simulink model "ATTN"  (R2023a)
settings: Solver=FixedStepAuto  StartTime=0.0  StopTime=40000  RelTol=1e-3
model workspace (MAT data in the model file):
  SampleTime = 0.001
  T_npxls = 4
  T_pupil = 100
  T_whisk = 20
  maxFrame = 3600000
  rewardDuration = 0.05
  targetSide = 1
  toneDuration = 1.5
  trainingStage = 3
  triangleAmplitude = 10
  triangleDuration = 0.1
undefined symbols (not defined in the file or in its folder): Ended, fdesignblkfcn, gcbh, Single
libraries: speedgoatlib_IO191 x5
(part 3 of 3)

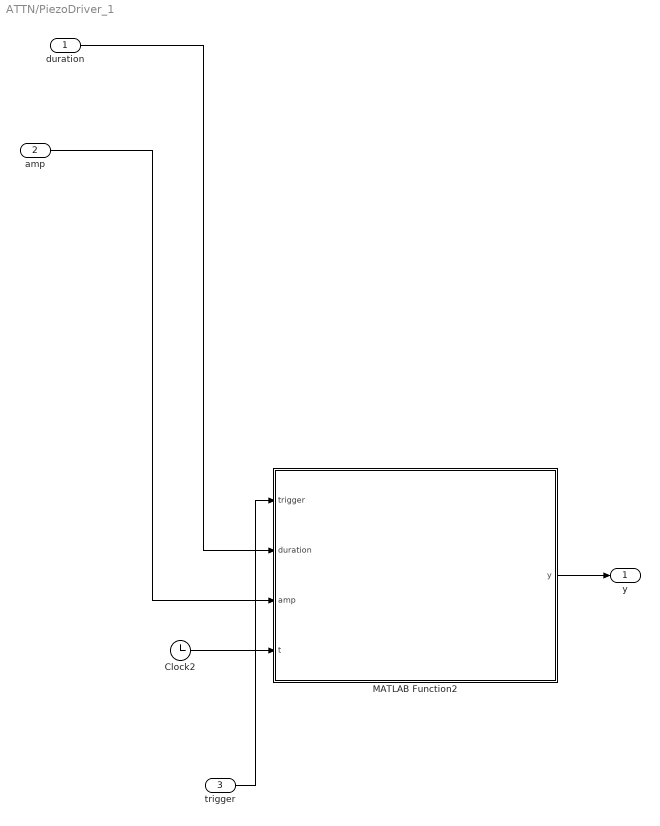
== system ATTN/PiezoDriver_1 ==
  duration : Inport
  amp : Inport  Port=2
  trigger : Inport  Port=3
  Clock2 : Clock
  MATLAB Function2 : MATLAB Function  TreatAsAtomicUnit=on
  y : Outport
  wires:
  Clock2/1 -> MATLAB Function2/4(t)
  MATLAB Function2/1(y) -> y/1
  amp/1 -> MATLAB Function2/3(amp)
  trigger/1 -> MATLAB Function2/1(trigger)
  duration/1 -> MATLAB Function2/2(duration)

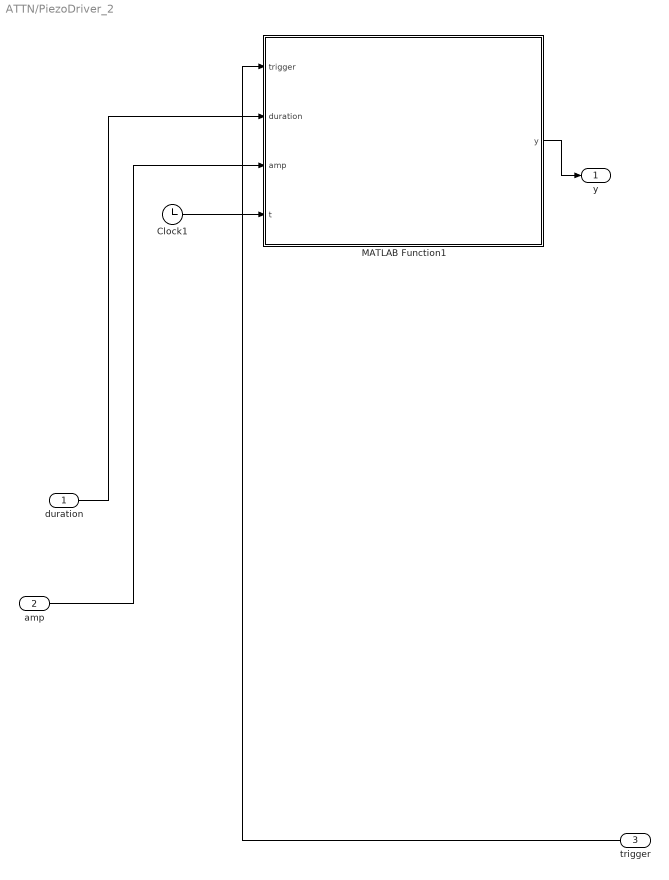
== system ATTN/PiezoDriver_2 ==
  duration : Inport
  amp : Inport  Port=2
  trigger : Inport  Port=3
  Clock1 : Clock
  MATLAB Function1 : MATLAB Function  TreatAsAtomicUnit=on
  y : Outport
  wires:
  Clock1/1 -> MATLAB Function1/4(t)
  trigger/1 -> MATLAB Function1/1(trigger)
  amp/1 -> MATLAB Function1/3(amp)
  duration/1 -> MATLAB Function1/2(duration)
  MATLAB Function1/1(y) -> y/1

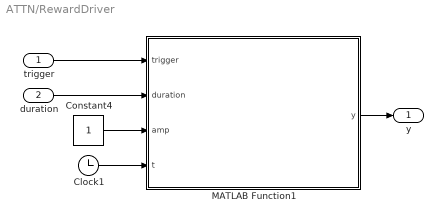
== system ATTN/RewardDriver ==
  trigger : Inport
  duration : Inport  Port=2
  Clock1 : Clock
  Constant4 : Constant  SampleTime=SampleTime
  MATLAB Function1 : MATLAB Function  TreatAsAtomicUnit=on
  y : Outport
  wires:
  Clock1/1 -> MATLAB Function1/4(t)
  Constant4/1 -> MATLAB Function1/3(amp)
  duration/1 -> MATLAB Function1/2(duration)
  trigger/1 -> MATLAB Function1/1(trigger)
  MATLAB Function1/1(y) -> y/1

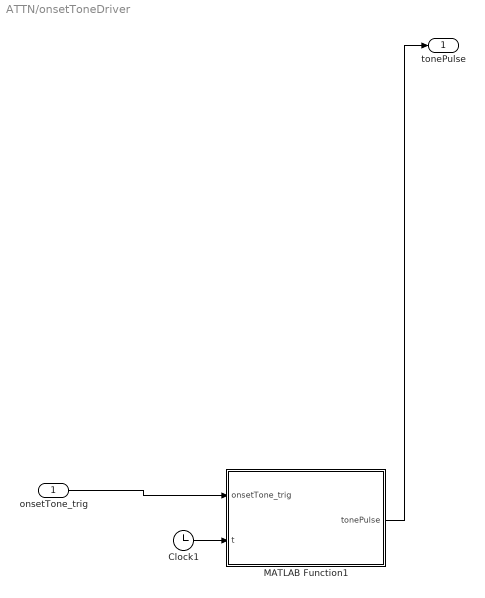
== system ATTN/onsetToneDriver ==
  onsetTone_trig : Inport
  Clock1 : Clock
  MATLAB Function1 : MATLAB Function  TreatAsAtomicUnit=on
  tonePulse : Outport
  wires:
  Clock1/1 -> MATLAB Function1/2(t)
  MATLAB Function1/1(tonePulse) -> tonePulse/1
  onsetTone_trig/1 -> MATLAB Function1/1(onsetTone_trig)

== matlab function ATTN/PiezoDriver_2/MATLAB Function1 ==
  data: trigger input; duration input; amp input; y output; t input
function y = drivePiezo(trigger, duration, amp, t) 
    % When the trigger is received, drivePiezo starts to output a triangle 
    % wave defined by duration and amplitude
    
    % If the trigger is not received, it checks whether t0 is not 
    % empty (indicating that a trigger has been received previously). 
    % If t0 is not empty, it checks if (t - t0) is less than 1.5 seconds. 
    % If so, it keeps tonePulse set to 1, maintaining the tone pulse for 
    % 1.5 seconds after the trigger. 
      
    
    persistent t0;
    persistent y0;
    increment = amp / (duration*1000/2);

    if trigger                
        t0 = t; % store current time 
        y = 0;
        y0 = y;
    elseif ~isempty(t0) 
        if (t - t0) <= duration/2
            y = y0 + increment;
            y0 = y;
        elseif (t - t0) <= duration
            y = y0 - increment;
            y = max([0,y]);
            y0 = y;
        else
            y = 0;
            clear t0 y0 % reset t0 to initial condition
        end        
    else % reset to 0 if no more trigger activity
        y = 0;        
    end

== matlab function ATTN/RewardDriver/MATLAB Function1 ==
  data: trigger input; y output; duration input; amp input; t input
function y = driveSpout(trigger, duration, amp, t) 
    % When the trigger is received, driveSpout starts to output a square
    % pulse defined by duration and amplitude
    
    % If the trigger is not received, it checks whether t0 is not 
    % empty (indicating that a trigger has been received previously). 
    % If t0 is not empty, it checks if (t - t0) is less than 1.5 seconds. 
    % If so, it keeps tonePulse set to 1, maintaining the tone pulse for 
    % 1.5 seconds after the trigger. 
      
    
    persistent t0;

    if trigger                     
        t0 = t; % store current time 
        y = amp;
    elseif ~isempty(t0) 
        if (t - t0) <= duration
            y = amp;
        else
            y = 0;
            clear t0 % reset t0 to initial condition
        end        
    else % reset to 0 if no more trigger activity
        y = 0;        
    end
end

== matlab function ATTN/MATLAB Function1 ==
  data: ADIn input; Lick output; y1 output; Thrd input; x1 input; x2 input; y2 output
function [Lick, y1, y2] = LickDetector(ADIn, Thrd, x1, x2)
%#codegen

ADIn = abs(ADIn);
if x1 == 0
    y1 = 0;
end


if ADIn > Thrd
    y1 = x1+1;
    y2 = x2;
else
    y1 = 0;
    y2 = 0;
end

if (y1 >20) && (x2 == 0)
    Lick =1;
    y2 = 1;
else
    Lick = 0;
%    y2 = x2;
end

== matlab function ATTN/MATLAB Function ==
  data: state_in input; localTime_in input; trialNum_in input; lick input; sessionTime input; npxlsAcq_in input; state_out output; localTime_out output; trialNum_out output; npxlsAcq_out output; counter_in input; numLicks_in input; delay_in input; right_trigger_in input; left_trigger_in input; sampleTime input; counter_out output; numLicks_out output; reward_trigger_out output; right_trigger_out output; left_trigger_out output; delay_out output; was_target_in input; was_target_out output; target_side input; reward_duration_in input; stim_duration_in input; stage input; reward_duration_out output; stim_duration_out output; onsetTone_trig output
function [state_out, localTime_out, trialNum_out, ...
    npxlsAcq_out, counter_out, numLicks_out, reward_trigger_out, ...
    right_trigger_out, left_trigger_out, delay_out, was_target_out, ... 
    reward_duration_out, stim_duration_out, onsetTone_trig] ...
    = nCORTEx(state_in, localTime_in, trialNum_in, lick, ...
    sessionTime, npxlsAcq_in, counter_in, numLicks_in, delay_in, ... 
    right_trigger_in, left_trigger_in, sampleTime, was_target_in, ...
    target_side, reward_duration_in, stim_duration_in, stage)
% stages: 1 - classical conditioning, 2 - opreant conditioning, 3 - impulse
% control, 111 - calibrate reward delivery; 222 - position piezo; 333 -
% calibrate piezo driver triangle duration 
    
    counter_out=counter_in+1;

    switch (stage)
        case {1} %% classical conditioning 
            switch (state_in)         
                % case {0} % LOAD SESSION PARAMS
                    % params = loadSlParams;
                    % state_out = 1;
                case {1} %% TRIAL START
                    npxlsAcq_out=1;
                    state_out = 2; % go to ITI
                    localTime_out = 1;
                    trialNum_out = 1;
                    % reset piezo triggers and lick counter
                    right_trigger_out = 0; % reset piezo triggers 
                    left_trigger_out = 0;
                    numLicks_out = 0;
                    delay_out = sessionTime + negative_exp_rand(5,9);
                    disp('End of ITI')
                    disp(delay_out)
                    reward_trigger_out = 0;
                    was_target_out = 0;
                    reward_duration_out = reward_duration_in;
                    stim_duration_out = stim_duration_in;
                    onsetTone_trig = 0;
        
                case {2} %% inter-trial interval  
                    if sessionTime < delay_in
                        state_out = state_in; % continue with ITI 
                    else
                        state_out = 3; % go to stimulus 
                    end
                    localTime_out = localTime_in + 1;
                    trialNum_out = trialNum_in + 1;
                    npxlsAcq_out=npxlsAcq_in;
                    right_trigger_out = right_trigger_in; % keep piezo triggers 
                    left_trigger_out = left_trigger_in;
                    numLicks_out = numLicks_in;
                    delay_out = delay_in;
                    reward_trigger_out = 0;
                    was_target_out = was_target_in;
                    reward_duration_out = reward_duration_in;
                    stim_duration_out = stim_duration_in;
                    onsetTone_trig = 0;
        
                case {3} %% stimulus onset 
                    if rand() <= 0.8 % 80% distractor stims 
                        if target_side % 1: left target
                            right_trigger_out = 1;
                            left_trigger_out = 0;
                        else % 0: right target
                            left_trigger_out = 1;
                            right_trigger_out = 0;
                        end
                        disp('Distractor')
                        disp(sessionTime)
                        was_target_out = 0;
                    else % 20% target stims 
                        if target_side % 1: left target
                            left_trigger_out = 1;
                            right_trigger_out = 0;
                        else
                            right_trigger_out = 1;
                            left_trigger_out = 0;
                        end
                        disp('Target')
                        disp(sessionTime)
                        was_target_out = 1;
                    end
                    % trigger a piezo  
                    state_out = 4; % go to lockout window
                    delay_out = sessionTime + 0.2;
                    disp('End of lockout')
                    disp(delay_out)
                    localTime_out = localTime_in + 1;
                    trialNum_out = trialNum_in + 1;
                    npxlsAcq_out=npxlsAcq_in;
                    numLicks_out = numLicks_in;
                    reward_trigger_out = 0;
                    reward_duration_out = reward_duration_in;
                    stim_duration_out = stim_duration_in;
                    onsetTone_trig = 0;
        
                case {4} %% lockout window 
                    if sessionTime < delay_in 
                        state_out = state_in;
                        delay_out = delay_in;
                    elseif was_target_in
                        state_out = 5; % deliver reward 
                        delay_out = sessionTime + 1.0;
                    else
                        state_out = 6; % jump to response window (unrewarded)
                        delay_out = sessionTime + 1.0;
                    end
                    localTime_out = localTime_in + 1;
                    trialNum_out = trialNum_in + 1;
                    npxlsAcq_out=npxlsAcq_in;
                    left_trigger_out = 0; % reset piezo triggers
                    right_trigger_out = 0;
                    numLicks_out = numLicks_in;
                    reward_trigger_out = 0;
                    was_target_out = was_target_in;
                    reward_duration_out = reward_duration_in;
                    stim_duration_out = stim_duration_in;
                    onsetTone_trig = 0;
             
                case {5} %% reward delivery `
                    % trigger reward 
                    reward_trigger_out = 1;
                    disp('Deliver Reward')
                    disp(sessionTime)
                    state_out = 6; % go to response window
                    delay_out = delay_in;
                    localTime_out = localTime_in + 1;
                    trialNum_out = trialNum_in + 1;
                    npxlsAcq_out=npxlsAcq_in;
                    numLicks_out = numLicks_in;
                    right_trigger_out = right_trigger_in;
                    left_trigger_out = left_trigger_in;
                    was_target_out = was_target_in;
                    reward_duration_out = reward_duration_in;
                    stim_duration_out = stim_duration_in;
                    onsetTone_trig = 0;

                case {6} %% response window 
                    if sessionTime < delay_in
                        state_out = state_in;
                    else
                        state_out = 1; % start new trial
                        disp('Start new trial')
                        disp(sessionTime)
                    end
                    localTime_out = localTime_in + 1;
                    trialNum_out = trialNum_in + 1;
                    npxlsAcq_out=npxlsAcq_in;
                    numLicks_out = numLicks_in;
                    right_trigger_out = right_trigger_in;
                    left_trigger_out = left_trigger_in;
                    delay_out = delay_in;
                    reward_trigger_out = 0;
                    was_target_out = was_target_in;
                    reward_duration_out = reward_duration_in;
                    stim_duration_out = stim_duration_in;
                    onsetTone_trig = 0;

                otherwise
                    state_out = state_in;
                    localTime_out = localTime_in;
                    trialNum_out = trialNum_in;
                    npxlsAcq_out=npxlsAcq_in;
                    right_trigger_out = right_trigger_in; % reset piezo triggers 
                    left_trigger_out = left_trigger_in;
                    numLicks_out = numLicks_in;
                    delay_out = delay_in;
                    reward_trigger_out = 0;
                    was_target_out = was_target_in;
                    reward_duration_out = reward_duration_in;
                    stim_duration_out = stim_duration_in;
                    onsetTone_trig = 0;
            end
        case {2} %% operant conditioning 
            switch (state_in)         
                % case {0} % LOAD SESSION PARAMS
                    % params = loadSlParams;
                    % state_out = 1;
                
                case {1} %% TRIAL START
                    npxlsAcq_out=1;
                    state_out = 2; % go to ITI
                    localTime_out = 1;
                    trialNum_out = 1;
                    % reset piezo triggers and lick counter
                    right_trigger_out = 0; % reset piezo triggers 
                    left_trigger_out = 0;
                    numLicks_out = 0;
                    delay_out = sessionTime + negative_exp_rand(5,9);
                    disp('End of ITI')
                    disp(delay_out)
                    reward_trigger_out = 0;
                    was_target_out = was_target_in;
                    reward_duration_out = reward_duration_in;
                    stim_duration_out = stim_duration_in;
                    onsetTone_trig = 0;

                case {2} %% inter-trial interval  
                    if sessionTime < delay_in
                        state_out = state_in; % continue with ITI 
                    else
                        state_out = 3; % go to stimulus 
                    end
                    localTime_out = localTime_in + 1;
                    trialNum_out = trialNum_in + 1;
                    npxlsAcq_out=npxlsAcq_in;
                    right_trigger_out = right_trigger_in; % keep piezo triggers 
                    left_trigger_out = left_trigger_in;
                    numLicks_out = numLicks_in;
                    delay_out = delay_in;
                    reward_trigger_out = 0;
                    was_target_out = was_target_in;
                    reward_duration_out = reward_duration_in;
                    stim_duration_out = stim_duration_in;
                    onsetTone_trig = 0;

                case {3} %% stimulus onset 
                    if rand() <= 0.8% distractor stims 
                        if target_side % 1: left target 
                            right_trigger_out = 1;
                            left_trigger_out = 0;
                        else % 0: right target 
                            left_trigger_out = 1;
                            right_trigger_out = 0;
                        end
                        disp('Distractor')
                        disp(sessionTime)
                        was_target_out = 0;
                    else % 20% target stims 
                        if target_side % 1: left target 
                            left_trigger_out = 1;
                            right_trigger_out = 0;
                        else % 0: right target 
                            right_trigger_out = 1;
                            left_trigger_out = 0;
                        end
                        disp('Target')
                        disp(sessionTime)
                        was_target_out = 1;
                    end
                    % trigger a piezo  
                    state_out = 4; % go to lockout window
                    delay_out = sessionTime + 0.2;
                    disp('End of lockout')
                    disp(delay_out)
                    localTime_out = localTime_in + 1;
                    trialNum_out = trialNum_in + 1;
                    npxlsAcq_out=npxlsAcq_in;
                    numLicks_out = numLicks_in;
                    reward_trigger_out = 0;
                    reward_duration_out = reward_duration_in;
                    stim_duration_out = stim_duration_in;
                    onsetTone_trig = 0;

                case {4} %% lockout window 
                    if sessionTime < delay_in 
                        state_out = state_in;
                        delay_out = delay_in;
                    else %if was_target_in
                        state_out = 5; % response window
                        delay_out = sessionTime + 1.5;
                    % else
                    %     state_out = 7; % jump to response window (unrewarded)
                    %     delay_out = sessionTime + 1.0;                   
                    end
                    localTime_out = localTime_in + 1;
                    trialNum_out = trialNum_in + 1;
                    npxlsAcq_out=npxlsAcq_in;
                    numLicks_out = numLicks_in;
                    reward_trigger_out = 0;
                    left_trigger_out = 0; % reset piezo targets 
                    right_trigger_out = 0;
                    was_target_out = was_target_in;
                    reward_duration_out = reward_duration_in;
                    stim_duration_out = stim_duration_in;
                    onsetTone_trig = 0;

                case {5} %% response window 
                    % increment numLicks based on lickometer input 
                    if lick
                        numLicks_out = numLicks_in + 1;
                    else
                        numLicks_out = numLicks_in;
                    end

                    if sessionTime < delay_in
                        state_out = state_in;
                    elseif numLicks_in && was_target_in
                        state_out = 6; % deliver reward
                    else
                        state_out = 1; % start new trial
                        disp('No response')
                        disp(left_trigger_in)
                    end
                    localTime_out = localTime_in + 1;
                    trialNum_out = trialNum_in + 1;
                    npxlsAcq_out=npxlsAcq_in;
                    right_trigger_out = right_trigger_in;
                    delay_out = delay_in;
                    reward_trigger_out = 0;
                    left_trigger_out = left_trigger_in;
                    was_target_out = was_target_in;
                    reward_duration_out = reward_duration_in;
                    stim_duration_out = stim_duration_in;
                    onsetTone_trig = 0;

                case {6} %% reward delivery 
                    % trigger reward 
                    reward_trigger_out = 1;
                    disp('Deliver Reward')
                    disp(sessionTime)
                    state_out = 7; % go to response window
                    delay_out = sessionTime + 0.5;
                    disp('Reward collection')
                    disp(delay_out)
                    localTime_out = localTime_in + 1;
                    trialNum_out = trialNum_in + 1;
                    npxlsAcq_out=npxlsAcq_in;
                    numLicks_out = numLicks_in;
                    right_trigger_out = right_trigger_in;
                    left_trigger_out = left_trigger_in;
                    was_target_out = was_target_in;
                    reward_duration_out = reward_duration_in;
                    stim_duration_out = stim_duration_in;
                    onsetTone_trig = 0;

                case {7} %% reward collection
                    if sessionTime < delay_in
                        state_out = state_in;
                    else
                        state_out = 1; %start new trial
                    end
                    localTime_out = localTime_in + 1;
                    trialNum_out = trialNum_in + 1;
                    npxlsAcq_out=npxlsAcq_in;
                    left_trigger_out = left_trigger_in;
                    right_trigger_out = right_trigger_in;
                    numLicks_out = numLicks_in;
                    delay_out = delay_in;
                    reward_trigger_out = 0;
                    was_target_out = was_target_in;
                    reward_duration_out = reward_duration_in;
                    stim_duration_out = stim_duration_in;
                    onsetTone_trig = 0;

                otherwise
                    state_out = state_in;
                    localTime_out = localTime_in;
                    trialNum_out = trialNum_in;
                    npxlsAcq_out=npxlsAcq_in;
                    left_trigger_out = left_trigger_in;
                    right_trigger_out = right_trigger_in;
                    numLicks_out = numLicks_in;
                    delay_out = delay_in;
                    reward_trigger_out = 0;
                    was_target_out = was_target_in;
                    reward_duration_out = reward_duration_in;
                    stim_duration_out = stim_duration_in;
                    onsetTone_trig = 0;
            end
        case {3} %% impulse control
            switch (state_in)         
                % case {0} % LOAD SESSION PARAMS
                    % params = loadSlParams;
                    % state_out = 1;
                case {1} %% TRIAL START
                    npxlsAcq_out=1;
                    state_out = 2; % go to ITI
                    localTime_out = 1;
                    trialNum_out = 1;
                    % reset piezo triggers and lick counter
                    right_trigger_out = 0; % reset piezo triggers 
                    left_trigger_out = 0;
                    if ~was_target_in && ~numLicks_in 
                        disp('CR')
                        delay_out = sessionTime + negative_exp_rand(2,4);
                    else
                        delay_out = sessionTime + negative_exp_rand(5,9);
                    end
                    numLicks_out = 0;
                    disp('End of ITI')
                    disp(delay_out)
                    reward_trigger_out = 0;
                    was_target_out = 0;
                    reward_duration_out = reward_duration_in;
                    stim_duration_out = stim_duration_in;
                    onsetTone_trig = 0;

                case {2} %% inter-trial interval  
                    if sessionTime < delay_in
                        state_out = state_in; % continue with ITI 
                    else
                        state_out = 3; % go to stimulus 
                    end
                    localTime_out = localTime_in + 1;
                    trialNum_out = trialNum_in + 1;
                    npxlsAcq_out=npxlsAcq_in;
                    right_trigger_out = right_trigger_in; % keep piezo triggers 
                    left_trigger_out = left_trigger_in;
                    numLicks_out = numLicks_in;
                    delay_out = delay_in;
                    reward_trigger_out = 0;
                    was_target_out = was_target_in;
                    reward_duration_out = reward_duration_in;
                    stim_duration_out = stim_duration_in;
                    onsetTone_trig = 0;

                case {3} %% stimulus onset 
                    if rand() <= 0.8 % 80% distractor stims 
                        if target_side % 1: target left
                            right_trigger_out = 1;
                            left_trigger_out = 0;
                        else % 0: target right
                            left_trigger_out = 1;
                            right_trigger_out = 0;
                        end
                        disp('Distractor')
                        disp(sessionTime)
                        was_target_out = 0;
                    else % 20% target stims 
                        if target_side % 1: target left
                            left_trigger_out = 1;
                            right_trigger_out = 0;
                        else % 0: target right
                            right_trigger_out = 1;
                            left_trigger_out = 0;
                        end
                        disp('Target')
                        disp(sessionTime)
                        was_target_out = 1;
                    end
                    % trigger a piezo  
                    state_out = 4; % go to lockout window
                    delay_out = sessionTime + 0.2;
                    disp('End of lockout')
                    disp(delay_out)
                    localTime_out = localTime_in + 1;
                    trialNum_out = trialNum_in + 1;
                    npxlsAcq_out=npxlsAcq_in;
                    numLicks_out = numLicks_in;
                    reward_trigger_out = 0;
                    reward_duration_out = reward_duration_in;
                    stim_duration_out = stim_duration_in;
                    onsetTone_trig = 0;

                case {4} %% lockout window 
                    if sessionTime < delay_in 
                        state_out = state_in;
                        delay_out = delay_in;
                    else %if was_target_in
                        state_out = 5; % response window
                        delay_out = sessionTime + 1.0;
                    % else
                    %     state_out = 7; % jump to response window (unrewarded)
                    %     delay_out = sessionTime + 1.0;                   
                    end
                    localTime_out = localTime_in + 1;
                    trialNum_out = trialNum_in + 1;
                    npxlsAcq_out=npxlsAcq_in;
                    numLicks_out = numLicks_in;
                    reward_trigger_out = 0;
                    left_trigger_out = 0;
                    right_trigger_out = 0;
                    was_target_out = was_target_in;
                    reward_duration_out = reward_duration_in;
                    stim_duration_out = stim_duration_in;
                    onsetTone_trig = 0;

                case {5} %% response window 
                    % increment numLicks based on lickometer input 
                    if was_target_in && rand() < 0.2
                        numLicks_out = numLicks_in + 1;
                    elseif ~was_target_in  && rand() < 0.001
                        numLicks_out = numLicks_in + 1;
                        disp('Licked for distractor')
                    else
                        numLicks_out = numLicks_in;
                    end

                    if sessionTime < delay_in
                        state_out = state_in;
                    elseif numLicks_in && was_target_in
                        state_out = 6; % deliver reward
                    else
                        state_out = 1; % start new trial
                        disp('No response')
                        disp(left_trigger_in)
                    end
                    localTime_out = localTime_in + 1;
                    trialNum_out = trialNum_in + 1;
                    npxlsAcq_out=npxlsAcq_in;
                    right_trigger_out = right_trigger_in;
                    delay_out = delay_in;
                    reward_trigger_out = 0;
                    left_trigger_out = left_trigger_in;
                    was_target_out = was_target_in;
                    reward_duration_out = reward_duration_in;
                    stim_duration_out = stim_duration_in;
                    onsetTone_trig = 0;

                case {6} %% reward delivery 
                    % trigger reward 
                    reward_trigger_out = 1;
                    disp('Deliver Reward')
                    disp(sessionTime)
                    state_out = 7; % go to response window
                    delay_out = sessionTime + 0.5;
                    disp('Reward collection')
                    disp(delay_out)
                    localTime_out = localTime_in + 1;
                    trialNum_out = trialNum_in + 1;
                    npxlsAcq_out=npxlsAcq_in;
                    numLicks_out = numLicks_in;
                    right_trigger_out = right_trigger_in;
                    left_trigger_out = left_trigger_in;
                    was_target_out = was_target_in;
                    reward_duration_out = reward_duration_in;
                    stim_duration_out = stim_duration_in;
                    onsetTone_trig = 0;

                case {7} %% reward collection
                    if sessionTime < delay_in
                        state_out = state_in;
                    else
                        state_out = 1; %start new trial
                    end
                    localTime_out = localTime_in + 1;
                    trialNum_out = trialNum_in + 1;
                    npxlsAcq_out=npxlsAcq_in;
                    left_trigger_out = left_trigger_in;
                    right_trigger_out = right_trigger_in;
                    numLicks_out = numLicks_in;
                    delay_out = delay_in;
                    reward_trigger_out = 0;
                    was_target_out = was_target_in;
                    reward_duration_out = reward_duration_in;
                    stim_duration_out = stim_duration_in;
                    onsetTone_trig = 0;

                otherwise
                    state_out = state_in;
                    localTime_out = localTime_in;
                    trialNum_out = trialNum_in;
                    npxlsAcq_out=npxlsAcq_in;
                    left_trigger_out = left_trigger_in;
                    right_trigger_out = right_trigger_in;
                    numLicks_out = numLicks_in;
                    delay_out = delay_in;
                    reward_trigger_out = 0;
                    was_target_out = was_target_in;
                    reward_duration_out = reward_duration_in;
                    stim_duration_out = stim_duration_in;
                    onsetTone_trig = 0;
            end
        case {111} % calibrate reward delivery 
            switch (state_in)         
                % case {0} % LOAD SESSION PARAMS
                    % params = loadSlParams;
                    % state_out = 1;
                case {1} %% TRIAL START
                    npxlsAcq_out=0;
                    localTime_out = 1;
                    trialNum_out = 1;
                    right_trigger_out = 0; % reset piezo triggers 
                    left_trigger_out = 0;
                    delay_out = sessionTime + 10;
                    numLicks_out = 0;
                    disp(sessionTime)
                    reward_trigger_out = 1;
                    was_target_out = 0;
                    reward_duration_out = 0.02;
                    disp(reward_duration_out)
                    state_out = 2; % go to ITI
                    stim_duration_out = stim_duration_in;
                    onsetTone_trig = 0;

                otherwise
                    if sessionTime < delay_in
                        state_out = state_in;
                        reward_trigger_out = 0;
                        delay_out = delay_in;
                        % reward_duration_out = (state_out-1) * 0.05;
                        reward_duration_out = 0.02;
                    else
                        state_out = state_in + 1; %start new trial
                        reward_trigger_out = 1;
                        delay_out = sessionTime + 10;
                        disp(sessionTime)
                        % reward_duration_out = state_out * 0.01;
                        reward_duration_out = 0.02;
                        disp(reward_duration_out)
                    end
                    localTime_out = localTime_in + 1;
                    trialNum_out = trialNum_in + 1;
                    npxlsAcq_out=npxlsAcq_in;
                    left_trigger_out = left_trigger_in;
                    right_trigger_out = right_trigger_in;
                    numLicks_out = numLicks_in;
                    was_target_out = was_target_in;
                    stim_duration_out = stim_duration_in;
                    onsetTone_trig = 0;
            end

        case {222} % piezo positioning, 1 target stim every 10 s
            switch (state_in)         
                % case {0} % LOAD SESSION PARAMS
                    % params = loadSlParams;
                    % state_out = 1;
                case {1} %% TRIAL START
                    npxlsAcq_out=0;
                    localTime_out = 1;
                    trialNum_out = 1;
                    if target_side % 1: target left
                        right_trigger_out = 1;
                        left_trigger_out = 0;
                    else % 0: target right
                        left_trigger_out = 1;
                        right_trigger_out = 0;
                    end
                    delay_out = sessionTime + 10;
                    numLicks_out = 0;
                    reward_trigger_out = 0;
                    was_target_out = 0;
                    reward_duration_out = reward_duration_in;
                    state_out = 2; % go to ITI
                    stim_duration_out = stim_duration_in;
                    onsetTone_trig = 0;
                    
                otherwise
                    if sessionTime < delay_in
                        state_out = state_in;
                        delay_out = delay_in;
                        left_trigger_out = 0;
                        right_trigger_out = 0;
                    else
                        state_out = state_in + 1; %start new trial
                        delay_out = sessionTime + 10;
                        if target_side % 1: target left
                            right_trigger_out = 1;
                            left_trigger_out = 0;
                        else % 0: target right
                            left_trigger_out = 1;
                            right_trigger_out = 0;
                        end
                    end
                    reward_trigger_out = 0;
                    localTime_out = localTime_in + 1;
                    trialNum_out = trialNum_in + 1;
                    npxlsAcq_out=npxlsAcq_in;
                    numLicks_out = numLicks_in;
                    was_target_out = was_target_in;
                    reward_duration_out = reward_duration_in;
                    stim_duration_out = stim_duration_in;
                    onsetTone_trig = 0;
                    
            end
        otherwise %case {333} % piezo calibration, 1 target stim every 10 s
            % incrememnt duration by 0.05
            switch (state_in)         
                % case {0} % LOAD SESSION PARAMS
                    % params = loadSlParams;
                    % state_out = 1;
                case {1} %% TRIAL START
                    npxlsAcq_out=0;
                    localTime_out = 1;
                    trialNum_out = 1;
                    if target_side % 1: target left
                        right_trigger_out = 1;
                        left_trigger_out = 0;
                    else % 0: target right
                        left_trigger_out = 1;
                        right_trigger_out = 0;
                    end
                    delay_out = sessionTime + 10;
                    numLicks_out = 0;
                    reward_trigger_out = 0;
                    was_target_out = 0;
                    stim_duration_out = 0.05;
                    state_out = 2; % go to ITI
                    reward_duration_out = reward_duration_in;
                    onsetTone_trig = 0;
                    
                otherwise
                    if sessionTime < delay_in
                        state_out = state_in;
                        delay_out = delay_in;
                        left_trigger_out = 0;
                        right_trigger_out = 0;
                        stim_duration_out = 0.05 * (state_in-1);
                    else
                        state_out = state_in + 1; %start new trial
                        delay_out = sessionTime + 10;
                        if target_side % 1: target left
                            right_trigger_out = 1;
                            left_trigger_out = 0;
                        else % 0: target right
                            left_trigger_out = 1;
                            right_trigger_out = 0;
                        end
                        stim_duration_out = 0.05 * state_in;
                    end
                    reward_trigger_out = 0;
                    localTime_out = localTime_in + 1;
                    trialNum_out = trialNum_in + 1;
                    npxlsAcq_out=npxlsAcq_in;
                    numLicks_out = numLicks_in;
                    was_target_out = was_target_in;
                    reward_duration_out = reward_duration_in;
                    onsetTone_trig = 0;
                   
            end
    end
    % if counter_out == tStop * 1000
    %     npxlsAcq_out = 0;
    % end
end

== matlab function ATTN/onsetToneDriver/MATLAB Function1 ==
  data: onsetTone_trig input; tonePulse output; t input
function tonePulse  = holdTone(onsetTone_trig, t) 
    % When the trigger onsetTone_trig is received, it sets tonePulse to 1 and 
    % stores the current time t in the persistent variable t0.   
    
    % If the trigger is not received (onsetTone_trig is false), it checks whether t0 is not 
    % empty (indicating that a trigger has been received previously). 
    % If t0 is not empty, it checks if (t - t0) is less than 1.5 seconds. 
    % If so, it keeps tonePulse set to 1, maintaining the tone pulse for 1.5 seconds after the trigger. 
    
    % After 1.5 seconds have passed since the trigger was received (when (t - t0) is 
    % greater than or equal to 1.5 seconds), it clears the persistent variable 
    % t0, effectively resetting it to its initial condition.     
    
    persistent t0;
    if onsetTone_trig                
        tonePulse = 1; % set tone pulse high until 1.5 s elapses            
        t0 = t; % store current time 
    elseif ~isempty(t0) 
        if (t - t0) < 1.5
            tonePulse = 1;
        else
            tonePulse = 0;
            clear t0 % reset t0 to initial condition
        end        
    else % reset to 0 if no more trigger activity
        tonePulse = 0;        
    end
end

== matlab function ATTN/PiezoDriver_1/MATLAB Function2 ==
  data: trigger input; duration input; amp input; y output; t input
function y = drivePiezo(trigger, duration, amp, t) 
    % When the trigger is received, drivePiezo starts to output a triangle 
    % wave defined by duration and amplitude
    
    % If the trigger is not received, it checks whether t0 is not 
    % empty (indicating that a trigger has been received previously). 
    % If t0 is not empty, it checks if (t - t0) is less than 1.5 seconds. 
    % If so, it keeps tonePulse set to 1, maintaining the tone pulse for 
    % 1.5 seconds after the trigger. 
      
    
    persistent t0;
    persistent y0;
    increment = amp / (duration*1000/2);

    if trigger                
        t0 = t; % store current time 
        y = 0;
        y0 = y;
    elseif ~isempty(t0) 
        if (t - t0) <= duration/2
            y = y0 + increment;
            y0 = y;
        elseif (t - t0) <= duration
            y = y0 - increment;
            y = max([0,y]);
            y0 = y;
        else
            y = 0;
            clear t0 y0 % reset t0 to initial condition
        end        
    else % reset to 0 if no more trigger activity
        y = 0;        
    end
